simulink model "mpc_switching"  (Simulink 7.4)
settings: Solver=ode45  SolverMode=SingleTasking  StartTime=0.0  StopTime=Tstop  FixedStep=1e-5  RelTol=1e-3
values from neighbouring files (symbols this model uses):
  b1 = 0.3    [mpcswitching.m]
  b2 = 0.8    [mpcswitching.m]
  k1 = 1    [mpcswitching.m]
  k2 = 0.1    [mpcswitching.m]
  M1 = 1    [mpcswitching.m]
  M2 = 5    [mpcswitching.m]    (also in mpctmpinit.m = 266.666666667)
  Ts = .05    (= 0.05)    [afti16.m]    (also in mpcbumpless.m = 0.5; mpccstr.m = 1; mpcdoubleint.m = 0.1; mpcmiso.m = 0.2)
  y1initial = 0    [mpcswitching.m]
  y2initial = 10    [mpcswitching.m]
  yeq1 = 10    [mpcswitching.m]
  yeq2 = -10    [mpcswitching.m]
libraries: simulink x4, mpclib x1
settings Model: Creator=jowen  LastModifiedBy=rchen  ExtModeTrigMode=oneshot  ExtModeArmWhenConnect=off
settings SolverCC: InsertRTBMode=Auto
settings DataIOCC: LimitDataPoints=off  SignalLoggingName=sigsOut
settings OptimizationCC: BooleanDataType=off  InlineInvariantSignals=on  InitFltsAndDblsToZero=on  EfficientMapNaN2IntZero=off
settings DebuggingCC: SaveWithParameterizedLinksMsg=none  CheckExecutionContextPreStartOutputMsg=on  CheckExecutionContextRuntimeOutputMsg=on  SignalResolutionControl=TryResolveAllWithWarning  SolverPrmCheckMsg=none  MultiTaskDSMMsg=warning  MultiTaskCondExecSysMsg=none  IntegerOverflowMsg=none  StrictBusMsg=None
settings HardwareCC: TargetEndianess=LittleEndian  TargetHWDeviceType=MATLAB Host  ProdEqTarget=off
settings RTWCC: IncludeERTFirstTime=on
settings GRTTargetCC: TargetFcnLib=ansi_tfl_tmw.mat

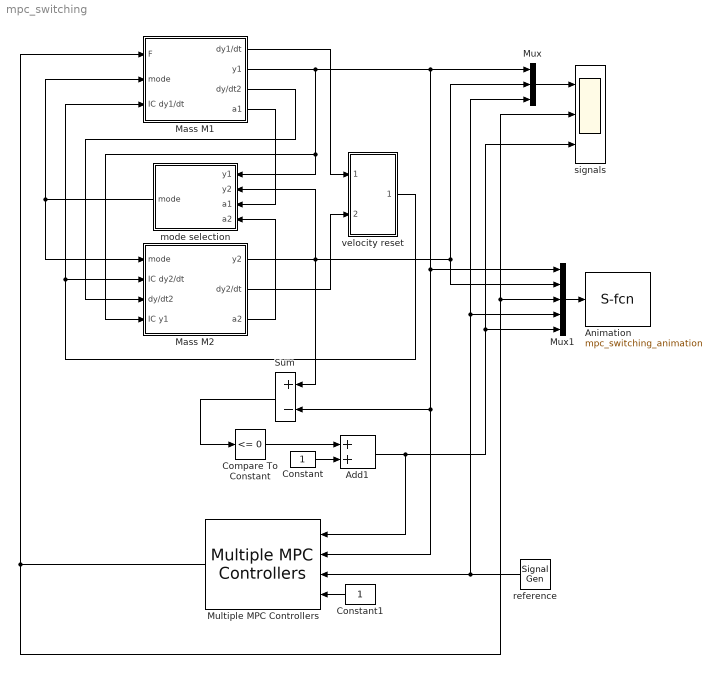
== system mpc_switching ==
  Add1 : Sum  OutDataType=sfix(16)  OutScaling=2^-10
  Animation : S-Function  FunctionName=mpc_switching_animation  Parameters=Ts,x0,speed,avifile,create_movie,yeq1,yeq2,OFF  EnableBusSupport=off  mask{x0=[y1initial;y2initial], speed=0.9, avifile='mpc_switching_demo', create_movie=off, OFF=false}
      mask prompts: x0 "Initial state"; speed "Animation speed, between 0 (slowest) and 1 (fastest)"; avifile "AVI file name for animation"; create_movie "Create AVI movie"; OFF "Animation Off"
      mask Display: image(double(imread('mpc_switching_spring.jpg'))/255);
  Compare To Constant : simulink/Logic and Bit Operations/Compare To Constant  SystemSampleTime=-1  relop=<=  const=0  LogicOutDataTypeMode=uint8  ZeroCross=off
  Constant : Constant  OutDataType=sfix(16)  OutScaling=2^0
  Constant1 : Constant  OutDataType=sfix(16)  OutScaling=2^0
  Mass M1 : Subsystem
  Mass M2 : Subsystem
  Multiple MPC Controllers : mpclib/Multiple MPC Controllers  SystemSampleTime=-1  Nmpc=2  theMPC=0  md_inport_multiple=on  mv_inport_multiple=off  lims_inport_multiple=off  mpcobjs={'MPC1','MPC2'}  x0s={'[]','[]'}  ref_signal_name_multiple=[]  ref_preview_multiple=on  ref_from_ws_multiple=off  md_signal_name_multiple=[]  md_preview_multiple=on  md_from_ws_multiple=off  nmv=0  linswitch=0
  Mux : Mux  Inputs=3
  Mux1 : Mux  Inputs=5
  Sum : Sum  Inputs=+-  OutDataType=sfix(16)  OutScaling=2^0
  mode selection : Subsystem
  reference : SignalGenerator  WaveForm=square  Amplitude=5  Frequency=.015
  signals : Scope  NumInputPorts=3
      settings: TimeRange=100  YMin=-10~0~0.5  YMax=10~25~2.5  DataFormat=Structure
  velocity reset : Subsystem
  wires:
  Mass M1/1(dy1/dt) -> velocity reset/1(dy1/dt)
  Mass M2/1(y2) -> mode selection/2(y2), Sum/1, Mux/2, Mux1/2
  Mass M1/2(y1) -> Mux/1, Sum/2, Multiple MPC Controllers/2, Mux1/1, mode selection/1(y1), Mass M2/4(IC y1)
  mode selection/1(mode) -> Mass M1/2(mode), Mass M2/1(mode)
  Mass M2/2(dy2/dt) -> velocity reset/2(dy2/dt)
  velocity reset/1(dy/dt) -> Mass M2/2(IC dy2/dt), Mass M1/3(IC dy1/dt)
  Mux/1 -> signals/1
  Constant/1 -> Add1/2
  Constant1/1 -> Multiple MPC Controllers/4
  Multiple MPC Controllers/1 -> Mass M1/1(F), Mux1/3, signals/2
  Mass M1/3(dy/dt2) -> Mass M2/3(dy/dt2)
  Add1/1 -> Mux1/5, signals/3, Multiple MPC Controllers/1
  reference/1 -> Mux/3, Mux1/4, Multiple MPC Controllers/3
  Mass M1/4(a1) -> mode selection/3(a1)
  Mass M2/3(a2) -> mode selection/4(a2)
  Compare To Constant/1 -> Add1/1
  Sum/1 -> Compare To Constant/1
  Mux1/1 -> Animation/1

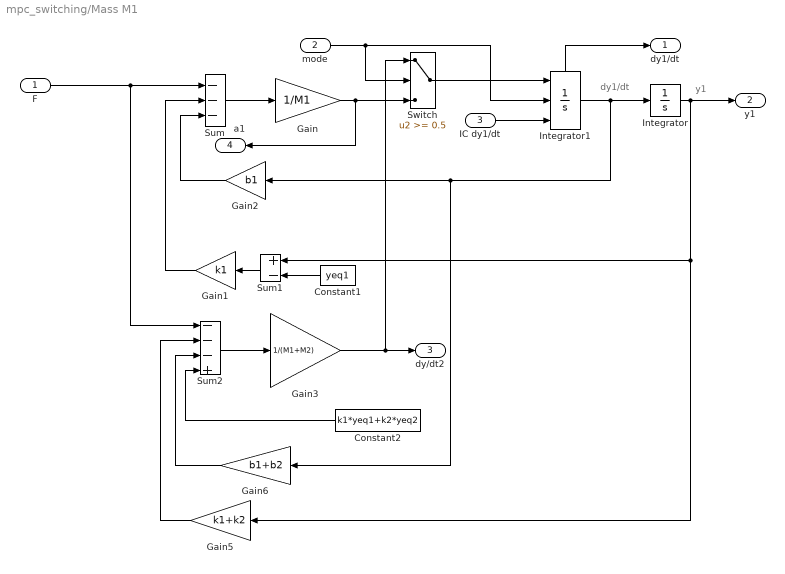
== system mpc_switching/Mass M1 ==
  note: y1
  note: dy1/dt
  F : Inport
  mode : Inport  Port=2
  IC dy1/dt : Inport  Port=3
  Constant1 : Constant  Value=yeq1  OutDataType=sfix(16)  OutScaling=2^0
  Constant2 : Constant  Value=k1*yeq1+k2*yeq2  OutDataType=sfix(16)  OutScaling=2^0
  Gain : Gain  Gain=1/M1  ParameterDataType=sfix(16)  ParameterScaling=2^0  OutDataType=sfix(16)  OutScaling=2^0
  Gain1 : Gain  Gain=k1  ParameterDataType=sfix(16)  ParameterScaling=2^0  OutDataType=sfix(16)  OutScaling=2^0
  Gain2 : Gain  Gain=b1  ParameterDataType=sfix(16)  ParameterScaling=2^0  OutDataType=sfix(16)  OutScaling=2^0
  Gain3 : Gain  Gain=1/(M1+M2)  ParameterDataType=sfix(16)  ParameterScaling=2^0  OutDataType=sfix(16)  OutScaling=2^0
  Gain5 : Gain  Gain=k1+k2  ParameterDataType=sfix(16)  ParameterScaling=2^0  OutDataType=sfix(16)  OutScaling=2^0
  Gain6 : Gain  Gain=b1+b2  ParameterDataType=sfix(16)  ParameterScaling=2^0  OutDataType=sfix(16)  OutScaling=2^0
  Integrator : Integrator  InitialCondition=y1initial
  Integrator1 : Integrator  ExternalReset=rising  InitialConditionSource=external  ShowStatePort=on
  Sum : Sum  Inputs=---  OutDataType=sfix(16)  OutScaling=2^0
  Sum1 : Sum  Inputs=+-  OutDataType=sfix(16)  OutScaling=2^0
  Sum2 : Sum  Inputs=---+  OutDataType=sfix(16)  OutScaling=2^0
  Switch : Switch  Threshold=0.5  OutDataType=sfix(16)  OutScaling=2^0
  dy1/dt : Outport
  y1 : Outport  Port=2
  dy/dt2 : Outport  Port=3
  a1 : Outport  Port=4
  wires:
  Integrator/1 -> Sum1/1, Gain5/1, y1/1
  Integrator1/1 -> Integrator/1, Gain2/1, Gain6/1
  Constant1/1 -> Sum1/2
  Sum1/1 -> Gain1/1
  Gain1/1 -> Sum/2
  Gain2/1 -> Sum/3
  F/1 -> Sum/1, Sum2/1
  mode/1 -> Integrator1/2, Switch/2
  Switch/1 -> Integrator1/1
  Sum/1 -> Gain/1
  Gain5/1 -> Sum2/2
  Gain6/1 -> Sum2/3
  Sum2/1 -> Gain3/1
  Constant2/1 -> Sum2/4
  Gain3/1 -> Switch/1, dy/dt2/1
  Gain/1 -> Switch/3, a1/1
  IC dy1/dt/1 -> Integrator1/3
  Integrator1/State -> dy1/dt/1

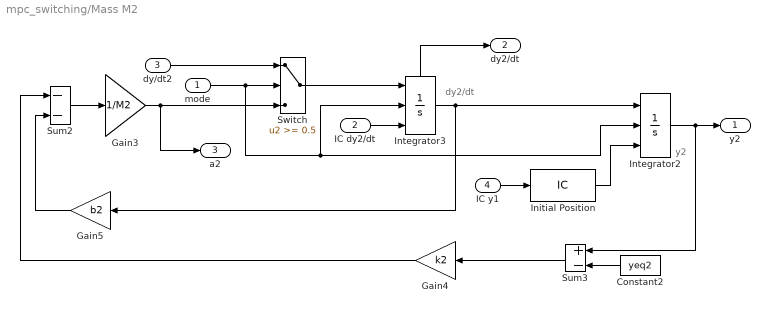
== system mpc_switching/Mass M2 ==
  note: dy2/dt
  note: y2
  mode : Inport
  IC dy2/dt : Inport  Port=2
  dy/dt2 : Inport  Port=3
  IC y1 : Inport  Port=4
  Constant2 : Constant  Value=yeq2  OutDataType=sfix(16)  OutScaling=2^0
  Gain3 : Gain  Gain=1/M2  ParameterDataType=sfix(16)  ParameterScaling=2^0  OutDataType=sfix(16)  OutScaling=2^0
  Gain4 : Gain  Gain=k2  ParameterDataType=sfix(16)  ParameterScaling=2^0  OutDataType=sfix(16)  OutScaling=2^0
  Gain5 : Gain  Gain=b2  ParameterDataType=sfix(16)  ParameterScaling=2^0  OutDataType=sfix(16)  OutScaling=2^0
  Initial Position : InitialCondition  Value=y2initial
  Integrator2 : Integrator  ExternalReset=rising  InitialConditionSource=external  InitialCondition=y2initial
  Integrator3 : Integrator  ExternalReset=rising  InitialConditionSource=external  ShowStatePort=on
  Sum2 : Sum  Inputs=--  OutDataType=sfix(16)  OutScaling=2^0
  Sum3 : Sum  Inputs=+-  OutDataType=sfix(16)  OutScaling=2^0
  Switch : Switch  Threshold=0.5  OutDataType=sfix(16)  OutScaling=2^0
  y2 : Outport
  dy2/dt : Outport  Port=2
  a2 : Outport  Port=3
  wires:
  Gain4/1 -> Sum2/1
  Gain5/1 -> Sum2/2
  Sum3/1 -> Gain4/1
  Constant2/1 -> Sum3/2
  Sum2/1 -> Gain3/1
  Integrator3/1 -> Gain5/1, Integrator2/1
  Integrator3/State -> dy2/dt/1
  Integrator2/1 -> Sum3/1, y2/1
  Switch/1 -> Integrator3/1
  mode/1 -> Integrator3/2, Integrator2/2, Switch/2
  Gain3/1 -> Switch/3, a2/1
  dy/dt2/1 -> Switch/1
  Initial Position/1 -> Integrator2/3
  IC y1/1 -> Initial Position/1
  IC dy2/dt/1 -> Integrator3/3

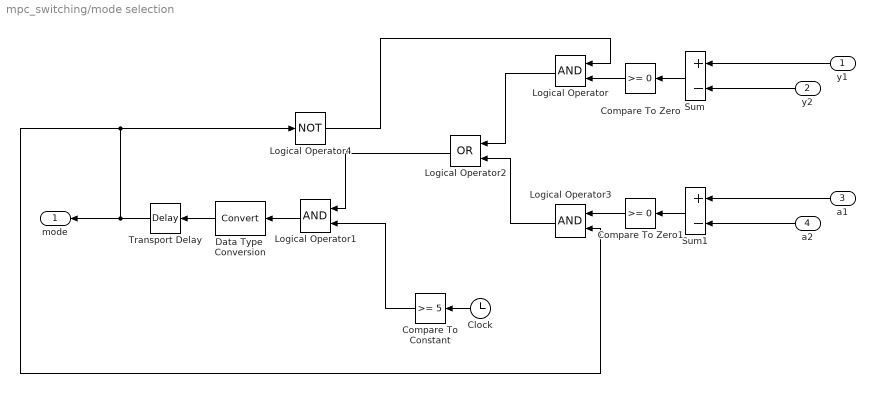
== system mpc_switching/mode selection ==
  y1 : Inport
  y2 : Inport  Port=2
  a1 : Inport  Port=3
  a2 : Inport  Port=4
  Clock : Clock
      settings: Decimation=10
  Compare To Constant : simulink/Logic and Bit Operations/Compare To Constant  SystemSampleTime=-1  relop=>=  const=5  LogicOutDataTypeMode=uint8  ZeroCross=off
  Compare To Zero : simulink/Logic and Bit Operations/Compare To Zero  SystemSampleTime=-1  relop=>=  LogicOutDataTypeMode=boolean  ZeroCross=off
  Compare To Zero1 : simulink/Logic and Bit Operations/Compare To Zero  SystemSampleTime=-1  relop=>=  LogicOutDataTypeMode=boolean  ZeroCross=off
  Data Type  Conversion : DataTypeConversion  OutDataType=sfix(16)  OutScaling=2^0
  Logical Operator : Logic  AllPortsSameDT=off  OutDataTypeMode=boolean  OutDataTypeStr=boolean
  Logical Operator1 : Logic  AllPortsSameDT=off  OutDataTypeMode=boolean  OutDataTypeStr=boolean
  Logical Operator2 : Logic  Operator=OR  AllPortsSameDT=off  OutDataTypeMode=boolean  OutDataTypeStr=boolean
  Logical Operator3 : Logic  AllPortsSameDT=off  OutDataTypeMode=boolean  OutDataTypeStr=boolean
  Logical Operator4 : Logic  Operator=NOT  AllPortsSameDT=off  OutDataTypeMode=boolean  OutDataTypeStr=boolean
  Sum : Sum  Inputs=+-  OutDataType=sfix(16)  OutScaling=2^0
  Sum1 : Sum  Inputs=+-  OutDataType=sfix(16)  OutScaling=2^0
  Transport Delay : TransportDelay  DelayTime=1e-6
  mode : Outport
  wires:
  y1/1 -> Sum/1
  y2/1 -> Sum/2
  Sum/1 -> Compare To Zero/1
  a1/1 -> Sum1/1
  a2/1 -> Sum1/2
  Sum1/1 -> Compare To Zero1/1
  Transport Delay/1 -> mode/1, Logical Operator3/2, Logical Operator4/1
  Logical Operator4/1 -> Logical Operator/1
  Compare To Zero/1 -> Logical Operator/2
  Logical Operator/1 -> Logical Operator2/1
  Logical Operator3/1 -> Logical Operator2/2
  Compare To Zero1/1 -> Logical Operator3/1
  Clock/1 -> Compare To Constant/1
  Logical Operator2/1 -> Logical Operator1/1
  Compare To Constant/1 -> Logical Operator1/2
  Logical Operator1/1 -> Data Type  Conversion/1
  Data Type  Conversion/1 -> Transport Delay/1

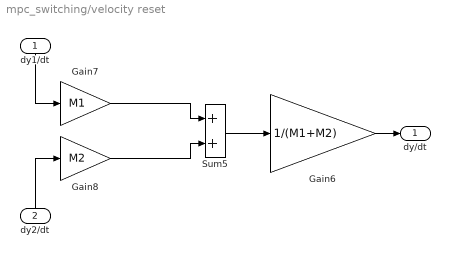
== system mpc_switching/velocity reset ==
  dy1/dt : Inport
  dy2/dt : Inport  Port=2
  Gain6 : Gain  Gain=1/(M1+M2)  ParameterDataType=sfix(16)  ParameterScaling=2^0  OutDataType=sfix(16)  OutScaling=2^0
  Gain7 : Gain  Gain=M1  ParameterDataType=sfix(16)  ParameterScaling=2^0  OutDataType=sfix(16)  OutScaling=2^0
  Gain8 : Gain  Gain=M2  ParameterDataType=sfix(16)  ParameterScaling=2^0  OutDataType=sfix(16)  OutScaling=2^0
  Sum5 : Sum  OutDataType=sfix(16)  OutScaling=2^0
  dy/dt : Outport
  wires:
  Sum5/1 -> Gain6/1
  Gain7/1 -> Sum5/1
  Gain8/1 -> Sum5/2
  dy1/dt/1 -> Gain7/1
  dy2/dt/1 -> Gain8/1
  Gain6/1 -> dy/dt/1
